simulink model "induction_machine_Simulink"  (Simulink 9.2)
settings: Solver=ode45  StartTime=0.0  StopTime=10.0  RelTol=1e-6  AbsTol=1e-8
values from neighbouring files (symbols this model uses):
  invL_matrix = inv(LMAT)    [IM_main_code.m]
  ir_alpha_0 = 0    [IM_main_code.m]
  ir_beta_0 = 0    [IM_main_code.m]
  is_alpha_0 = 0    [IM_main_code.m]
  is_beta_0 = 0    [IM_main_code.m]
  J = 0.05    [IM_main_code.m]
  Lm = 0.132    [IM_main_code.m]
  Lr = Lrl+Lm    (= 0.14006)    [IM_main_code.m]
  np = 2    [IM_main_code.m]
  Rr = 1.327    [IM_main_code.m]
  Rs = 1.33    [IM_main_code.m]
  theta0 = Us_theta0    [IM_main_code.m]
  thetar_0 = 0    [IM_main_code.m]
  ustep1 = Uspeak    [IM_main_code.m]
  ustep_time1 = Us_step_time    [IM_main_code.m]
  wr_0 = 0    [IM_main_code.m]
  ws = wslab    [IM_main_code.m]    (also in Post_Pross.m)
undefined symbols (not defined in the file or in its folder): j
settings Model: Creator=e6zebra  LastModifiedBy=e6zebra  ExtModeTrigMode=oneshot  ExtModeArmWhenConnect=off  ExtModeAutoUpdateStatusClock=off
settings SolverCC: AutoScaleAbsTol=off
settings DataIOCC: LimitDataPoints=off
settings OptimizationCC: BlockReduction=off  BooleanDataType=off  ExpressionDepthLimit=2147483647  InitFltsAndDblsToZero=on
settings DebuggingCC: SaveWithParameterizedLinksMsg=none  SignalResolutionControl=TryResolveAllWithWarning  MultiTaskDSMMsg=warning  MultiTaskCondExecSysMsg=none
settings HardwareCC: TargetUnknown=on
settings RTWCC: TemplateMakefile=grt.tmf
settings GRTTargetCC: TargetFcnLib=ansi_tfl_tmw.mat

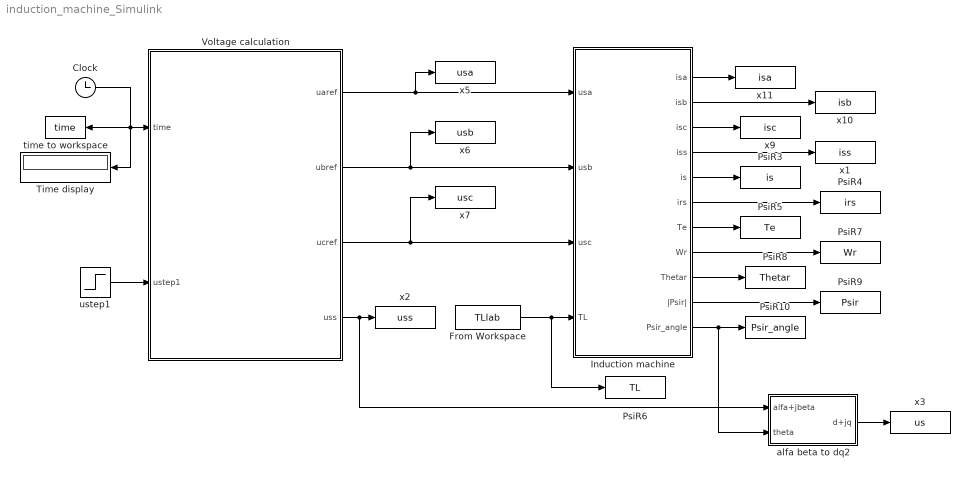
== system induction_machine_Simulink ==
  Clock : Clock
  From Workspace : FromWorkspace  VariableName=TLlab  SampleTime=0
  Induction machine : Subsystem
  PsiR10 : ToWorkspace  VariableName=Psir_angle  SampleTime=-1
  PsiR3 : ToWorkspace  VariableName=is  SampleTime=-1
  PsiR4 : ToWorkspace  VariableName=irs  SampleTime=-1
  PsiR5 : ToWorkspace  VariableName=Te  SampleTime=-1
  PsiR6 : ToWorkspace  VariableName=TL  SampleTime=-1
  PsiR7 : ToWorkspace  VariableName=Wr  SampleTime=-1
  PsiR8 : ToWorkspace  VariableName=Thetar  SampleTime=-1
  PsiR9 : ToWorkspace  VariableName=Psir  SampleTime=-1
  Time display : Display
  Voltage calculation : Subsystem
  alfa beta to dq2 : Subsystem
  time to workspace : ToWorkspace  VariableName=time  SampleTime=-1
  ustep1 : Step  Time=ustep_time1  After=ustep1  SampleTime=0
  x1 : ToWorkspace  VariableName=iss  SampleTime=-1
  x10 : ToWorkspace  VariableName=isb  SampleTime=-1
  x11 : ToWorkspace  VariableName=isa  SampleTime=-1
  x2 : ToWorkspace  VariableName=uss  SampleTime=-1
  x3 : ToWorkspace  VariableName=us  SampleTime=-1
  x5 : ToWorkspace  VariableName=usa  SampleTime=-1
  x6 : ToWorkspace  VariableName=usb  SampleTime=-1
  x7 : ToWorkspace  VariableName=usc  SampleTime=-1
  x9 : ToWorkspace  VariableName=isc  SampleTime=-1
  wires:
  Clock/1 -> Time display/1, time to workspace/1, Voltage calculation/1(time)
  Voltage calculation/1(uaref) -> x5/1, Induction machine/1(usa)
  Voltage calculation/2(ubref) -> x6/1, Induction machine/2(usb)
  Voltage calculation/3(ucref) -> x7/1, Induction machine/3(usc)
  ustep1/1 -> Voltage calculation/2(ustep1)
  Induction machine/4(iss) -> x1/1
  Induction machine/5(is) -> PsiR3/1
  Induction machine/7(Te) -> PsiR5/1
  Induction machine/6(irs) -> PsiR4/1
  Induction machine/8(Wr) -> PsiR7/1
  Induction machine/10(|Psir|) -> PsiR9/1
  Induction machine/9(Thetar) -> PsiR8/1
  Induction machine/11(Psir_angle) -> alfa beta to dq2/2(theta), PsiR10/1
  Induction machine/3(isc) -> x9/1
  Induction machine/2(isb) -> x10/1
  Induction machine/1(isa) -> x11/1
  From Workspace/1 -> Induction machine/4(TL), PsiR6/1
  Voltage calculation/4(uss) -> alfa beta to dq2/1(alfa+jbeta), x2/1
  alfa beta to dq2/1(d+jq) -> x3/1

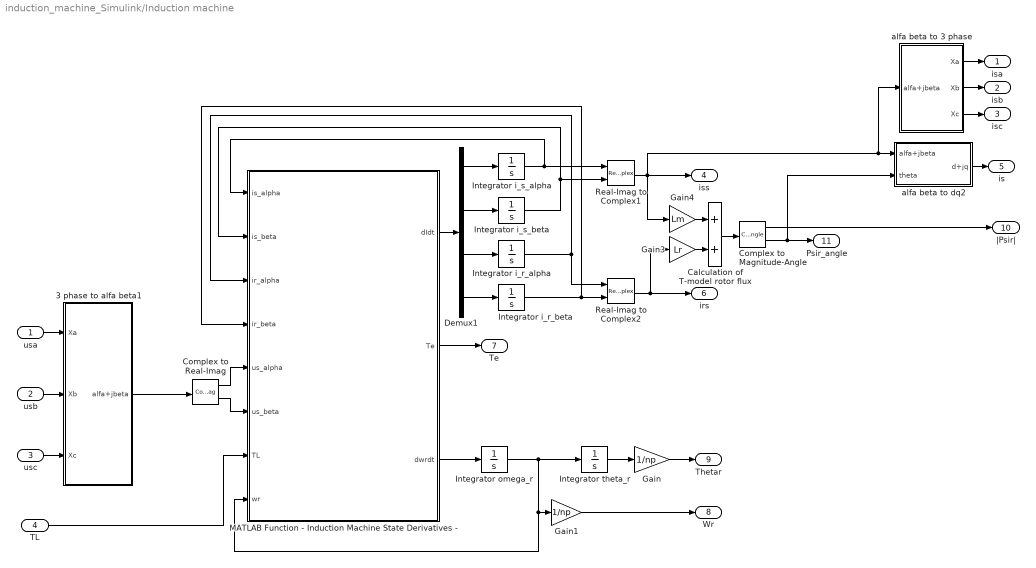
== system induction_machine_Simulink/Induction machine ==
  usa : Inport
  usb : Inport  Port=2
  usc : Inport  Port=3
  TL : Inport  Port=4
  3 phase to alfa beta1 : Subsystem
  Calculation of T-model rotor flux : Sum  SaturateOnIntegerOverflow=on  InputSameDT=on  OutDataTypeStr=Inherit: Same as first input
  Complex to Magnitude-Angle : ComplexToMagnitudeAngle
  Complex to Real-Imag : ComplexToRealImag
  Demux1 : Demux
  Gain : Gain  Gain=1/np
  Gain1 : Gain  Gain=1/np
  Gain3 : Gain  Gain=Lr
  Gain4 : Gain  Gain=Lm
  Integrator i_r_alpha : Integrator  InitialCondition=ir_alpha_0
  Integrator i_r_beta : Integrator  InitialCondition=ir_beta_0
  Integrator i_s_alpha : Integrator  InitialCondition=is_alpha_0
  Integrator i_s_beta : Integrator  InitialCondition=is_beta_0
  Integrator omega_r : Integrator  InitialCondition=wr_0
  Integrator theta_r : Integrator  InitialCondition=thetar_0
  MATLAB Function - Induction Machine State Derivatives - : MATLAB Function  TreatAsAtomicUnit=on
  Real-Imag to Complex1 : RealImagToComplex
  Real-Imag to Complex2 : RealImagToComplex
  alfa beta to 3 phase : Subsystem
  alfa beta to dq2 : Subsystem
  isa : Outport
  isb : Outport  Port=2
  isc : Outport  Port=3
  iss : Outport  Port=4
  is : Outport  Port=5
  irs : Outport  Port=6
  Te : Outport  Port=7
  Wr : Outport  Port=8
  Thetar : Outport  Port=9
  |Psir| : Outport  Port=10
  Psir_angle : Outport  Port=11
  wires:
  TL/1 -> MATLAB Function - Induction Machine State Derivatives -/7(TL)
  Real-Imag to Complex1/1 -> Gain4/1, iss/1, alfa beta to dq2/1(alfa+jbeta), alfa beta to 3 phase/1(alfa+jbeta)
  alfa beta to dq2/1(d+jq) -> is/1
  Real-Imag to Complex2/1 -> Gain3/1, irs/1
  Complex to Magnitude-Angle/1 -> |Psir|/1
  3 phase to alfa beta1/1(alfa+jbeta) -> Complex to Real-Imag/1
  usc/1 -> 3 phase to alfa beta1/3(Xc)
  usb/1 -> 3 phase to alfa beta1/2(Xb)
  usa/1 -> 3 phase to alfa beta1/1(Xa)
  alfa beta to 3 phase/1(Xa) -> isa/1
  alfa beta to 3 phase/3(Xc) -> isc/1
  alfa beta to 3 phase/2(Xb) -> isb/1
  Demux1/2 -> Integrator i_s_beta/1
  Demux1/3 -> Integrator i_r_alpha/1
  Demux1/4 -> Integrator i_r_beta/1
  Demux1/1 -> Integrator i_s_alpha/1
  MATLAB Function - Induction Machine State Derivatives -/1(dIdt) -> Demux1/1
  Integrator omega_r/1 -> Integrator theta_r/1, Gain1/1, MATLAB Function - Induction Machine State Derivatives -/8(wr)
  MATLAB Function - Induction Machine State Derivatives -/3(dwrdt) -> Integrator omega_r/1
  Integrator i_s_alpha/1 -> Real-Imag to Complex1/1, MATLAB Function - Induction Machine State Derivatives -/1(is_alpha)
  Integrator i_s_beta/1 -> Real-Imag to Complex1/2, MATLAB Function - Induction Machine State Derivatives -/2(is_beta)
  Integrator i_r_alpha/1 -> Real-Imag to Complex2/1, MATLAB Function - Induction Machine State Derivatives -/3(ir_alpha)
  Integrator i_r_beta/1 -> MATLAB Function - Induction Machine State Derivatives -/4(ir_beta), Real-Imag to Complex2/2
  Complex to Real-Imag/1 -> MATLAB Function - Induction Machine State Derivatives -/5(us_alpha)
  Complex to Real-Imag/2 -> MATLAB Function - Induction Machine State Derivatives -/6(us_beta)
  Integrator theta_r/1 -> Gain/1
  Gain/1 -> Thetar/1
  Gain1/1 -> Wr/1
  MATLAB Function - Induction Machine State Derivatives -/2(Te) -> Te/1
  Calculation of T-model rotor flux/1 -> Complex to Magnitude-Angle/1
  Complex to Magnitude-Angle/2 -> alfa beta to dq2/2(theta), Psir_angle/1
  Gain3/1 -> Calculation of T-model rotor flux/2
  Gain4/1 -> Calculation of T-model rotor flux/1

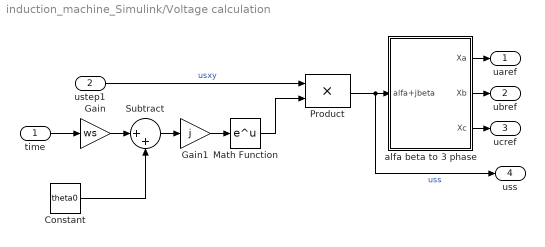
== system induction_machine_Simulink/Voltage calculation ==
  time : Inport
  ustep1 : Inport  Port=2
  Constant : Constant  Value=theta0
  Gain : Gain  Gain=ws
  Gain1 : Gain  Gain=j  SaturateOnIntegerOverflow=on  OutDataTypeStr=Inherit: Same as input  ParamDataTypeStr=Inherit: Same as input
  Math Function : Math  SaturateOnIntegerOverflow=on
  Product : Product  SaturateOnIntegerOverflow=on  OutDataTypeStr=Inherit: Same as first input
  Subtract : Sum  Inputs=|++
  alfa beta to 3 phase : Subsystem
  uaref : Outport
  ubref : Outport  Port=2
  ucref : Outport  Port=3
  uss : Outport  Port=4
  wires:
  time/1 -> Gain/1
  alfa beta to 3 phase/1(Xa) -> uaref/1
  alfa beta to 3 phase/2(Xb) -> ubref/1
  alfa beta to 3 phase/3(Xc) -> ucref/1
  ustep1/1 -> Product/1  "usxy"
  Gain1/1 -> Math Function/1
  Math Function/1 -> Product/2
  Product/1 -> alfa beta to 3 phase/1(alfa+jbeta), uss/1  "uss"
  Subtract/1 -> Gain1/1
  Gain/1 -> Subtract/1
  Constant/1 -> Subtract/2

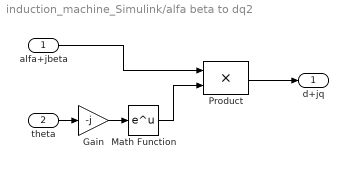
== system induction_machine_Simulink/alfa beta to dq2 ==
  alfa+jbeta : Inport
  theta : Inport  Port=2
  Gain : Gain  Gain=-j  SaturateOnIntegerOverflow=on  OutDataTypeStr=Inherit: Same as input  ParamDataTypeStr=Inherit: Same as input
  Math Function : Math  SaturateOnIntegerOverflow=on
  Product : Product  SaturateOnIntegerOverflow=on  OutDataTypeStr=Inherit: Same as first input
  d+jq : Outport
  wires:
  theta/1 -> Gain/1
  Gain/1 -> Math Function/1
  Math Function/1 -> Product/2
  alfa+jbeta/1 -> Product/1
  Product/1 -> d+jq/1

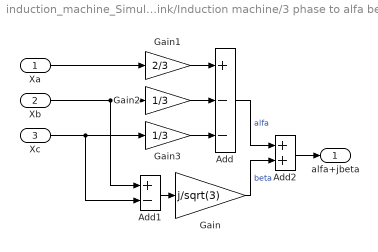
== system induction_machine_Simulink/Induction machine/3 phase to alfa beta1 ==
  Xa : Inport
  Xb : Inport  Port=2
  Xc : Inport  Port=3
  Add : Sum  Inputs=+--
  Add1 : Sum  Inputs=+-
  Add2 : Sum
  Gain : Gain  Gain=j/sqrt(3)
  Gain1 : Gain  Gain=2/3
  Gain2 : Gain  Gain=1/3
  Gain3 : Gain  Gain=1/3
  alfa+jbeta : Outport
  wires:
  Add1/1 -> Gain/1
  Add2/1 -> alfa+jbeta/1
  Gain/1 -> Add2/2  "beta"
  Add/1 -> Add2/1  "alfa"
  Gain3/1 -> Add/3
  Gain2/1 -> Add/2
  Gain1/1 -> Add/1
  Xa/1 -> Gain1/1
  Xb/1 -> Gain2/1, Add1/1
  Xc/1 -> Gain3/1, Add1/2

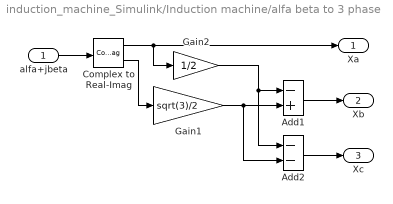
== system induction_machine_Simulink/Induction machine/alfa beta to 3 phase ==
  alfa+jbeta : Inport
  Add1 : Sum  Inputs=-+
  Add2 : Sum  Inputs=--
  Complex to Real-Imag : ComplexToRealImag
  Gain1 : Gain  Gain=sqrt(3)/2
  Gain2 : Gain  Gain=1/2
  Xa : Outport
  Xb : Outport  Port=2
  Xc : Outport  Port=3
  wires:
  alfa+jbeta/1 -> Complex to Real-Imag/1
  Complex to Real-Imag/1 -> Xa/1, Gain2/1
  Add2/1 -> Xc/1
  Add1/1 -> Xb/1
  Complex to Real-Imag/2 -> Gain1/1
  Gain1/1 -> Add1/2, Add2/2
  Gain2/1 -> Add1/1, Add2/1

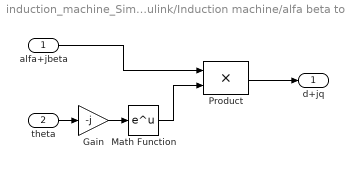
== system induction_machine_Simulink/Induction machine/alfa beta to dq2 ==
  alfa+jbeta : Inport
  theta : Inport  Port=2
  Gain : Gain  Gain=-j  SaturateOnIntegerOverflow=on  OutDataTypeStr=Inherit: Same as input  ParamDataTypeStr=Inherit: Same as input
  Math Function : Math  SaturateOnIntegerOverflow=on
  Product : Product  SaturateOnIntegerOverflow=on  OutDataTypeStr=Inherit: Same as first input
  d+jq : Outport
  wires:
  theta/1 -> Gain/1
  Gain/1 -> Math Function/1
  Math Function/1 -> Product/2
  alfa+jbeta/1 -> Product/1
  Product/1 -> d+jq/1

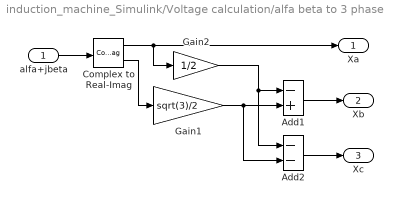
== system induction_machine_Simulink/Voltage calculation/alfa beta to 3 phase ==
  alfa+jbeta : Inport
  Add1 : Sum  Inputs=-+
  Add2 : Sum  Inputs=--
  Complex to Real-Imag : ComplexToRealImag
  Gain1 : Gain  Gain=sqrt(3)/2
  Gain2 : Gain  Gain=1/2
  Xa : Outport
  Xb : Outport  Port=2
  Xc : Outport  Port=3
  wires:
  alfa+jbeta/1 -> Complex to Real-Imag/1
  Complex to Real-Imag/1 -> Xa/1, Gain2/1
  Add2/1 -> Xc/1
  Add1/1 -> Xb/1
  Complex to Real-Imag/2 -> Gain1/1
  Gain1/1 -> Add1/2, Add2/2
  Gain2/1 -> Add1/1, Add2/1

== matlab function Induction machine/MATLAB Function - Induction Machine State Derivatives - ==
  data: is_alpha input double; is_beta input double; ir_alpha input double; ir_beta input double; us_alpha input double; us_beta input double; TL input double; dIdt output double size=4; Te output double size=1; dwrdt output double size=1; wr input double; np parameter double; Rs parameter double; Rr parameter double; invL_matrix parameter double; Lr parameter double; Lm parameter double; J parameter double
function [ dIdt , Te, dwrdt ] = induction_machine_state_derivatives( is_alpha , is_beta, ir_alpha , ir_beta , us_alpha , us_beta , TL , wr , np , Rs , Rr , invL_matrix , Lr , Lm , J)
% Description
% Standard syntax of funtion in MATLAB:
% funtion [ function_outputs ] =function_name( function_inputs )
% Use the same variable names as given in the inputs and outputs of the function

%%%%%%%%%%%%%%%%%%%%%%%%%%%%%%%%%%%%%%%%
% Calculating the electrical Derivatives

% Defining the resistance matrix RMAT
RMAT=[Rs,0,0,0;
	0,Rs,0,0;
	0,wr*Lm,Rr,wr*Lr;
	-wr*Lm,0,-wr*Lr,Rr];

% Defining the current and voltage vectors
I_vector = [ is_alpha ; is_beta ; ir_alpha ; ir_beta ];
U_vector = [ us_alpha ; us_beta ;        0 ;       0 ];

% Calculating the 4 current derivatives
dIdt = -invL_matrix*RMAT * I_vector + invL_matrix*U_vector;

%%%%%%%%%%%%%%%%%%%%%%%%%%%%%%%%%%%%%%%%
% Calculating the Mechanical Derivatives

% Calculating the electrodynamical torque
Te=3*np/2*Lm*(ir_alpha*is_beta-is_alpha*ir_beta);

%  Calculating the rotor speed derivative  
dwrdt=np/J*(Te-TL);

end
